simulink model "HW_2_Block_Diagram"  (R2023b)
settings: Solver=VariableStepAuto  StartTime=0.0  StopTime=15  RelTol=1e-3
values from neighbouring files (symbols this model uses):
  b = 100    [HW_2.mat]    (also in HW_2_a_Rev_1.m)
  gamma = 1    [HW_2.mat]    (also in HW_2_a_Rev_1.m)
settings Model: Creator=hkurt  LastModifiedBy=hkurt

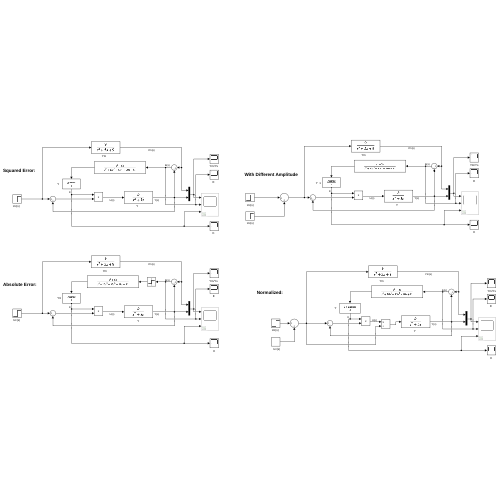
[thumbnail: Simulink's stored preview of the top-level diagram]
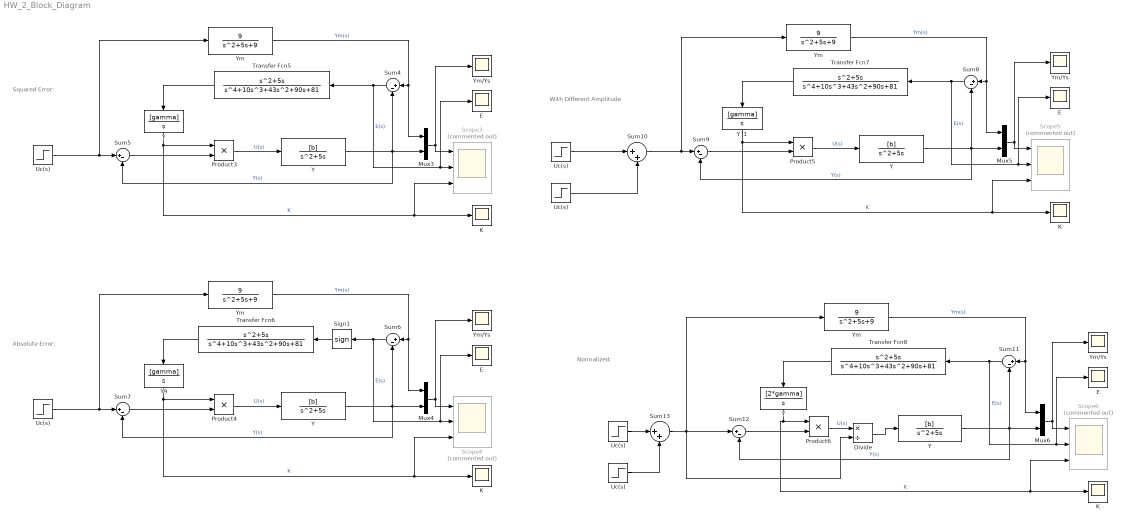
== system HW_2_Block_Diagram ==
  note: Squared Error:
  note: Absolute Error:
  note: With Different Amplitude
  note: Normalized:
  "          Uc(s)       " : Step  Time=5  After=4  SampleTime=0
  "         Uc(s)        " : Step  Time=5  After=3  SampleTime=0
  "  K  " : Scope
  "  Ym/Ys " : Scope
  " E " : Scope
  " E  " : Scope
  " K " : Scope
  " Uc(s)" : Step  SampleTime=0
  " Uc(s)  " : Step  Time=0  SampleTime=0
  " Y  " : TransferFcn  Numerator=[2*gamma]  Denominator=[1 0]
  " Y   " : TransferFcn  Numerator=[b]  Denominator=[1 5 0]
  " Ym    " : TransferFcn  Numerator=[9]  Denominator=[1 5 9]
  " Ym/Ys " : Scope
  Divide : Product  Inputs=*/
  "E " : Scope
  "E  " : Scope
  K : Scope
  "K  " : Scope
  Mux{3..6} (4 alike) : Mux  Inputs=2
  Product{3..6} (4 alike) : Product
  Scope{3..6} (4 alike) : Scope  Commented=on  NumInputPorts=3
  Sign1 : Signum
  Sum10 : Sum  Inputs=|++
  Sum{4..9,11..12} (8 alike) : Sum  Inputs=|+-
  Sum13 : Sum  Inputs=|++
  Transfer Fcn{5..8} (4 alike) : TransferFcn  Numerator=[1 5 0]  Denominator=[1 10 43 90 81]
  "Uc(s) " : Step  SampleTime=0
  "Uc(s)  " : Step  SampleTime=0
  "Y " : TransferFcn  Numerator=[b]  Denominator=[1 5 0]
  "Y  " : TransferFcn  Numerator=[gamma]  Denominator=[1 0]
  "Y   " : TransferFcn  Numerator=[b]  Denominator=[1 5 0]
  "Y    " : TransferFcn  Numerator=[b]  Denominator=[1 5 0]
  Y  1 : TransferFcn  Numerator=[gamma]  Denominator=[1 0]
  Y9 : TransferFcn  Numerator=[gamma]  Denominator=[1 0]
  "Ym  " : TransferFcn  Numerator=[9]  Denominator=[1 5 9]
  "Ym    " : TransferFcn  Numerator=[9]  Denominator=[1 5 9]
  "Ym     " : TransferFcn  Numerator=[9]  Denominator=[1 5 9]
  "Ym/Ys " : Scope
  "Ym/Ys  " : Scope
  wires:
  Mux3/1 -> "Ym/Ys "/1, Scope3/1
  "Y   "/1 -> Sum4/2, Mux3/2, Sum5/2  "Y(s)"
  Sum4/1 -> Transfer Fcn5/1, "E  "/1, Scope3/2  "E(s)"
  Transfer Fcn5/1 -> "Y  "/1
  "Y  "/1 -> "K  "/1, Scope3/3, Product3/1  "K"
  Product3/1 -> "Y   "/1  "U(s)"
  "Ym    "/1 -> Mux3/1, Sum4/1  "Ym(s)"
  Sum5/1 -> Product3/2
  "Uc(s)  "/1 -> Sum5/1, "Ym    "/1
  Mux4/1 -> "Ym/Ys  "/1, Scope4/1
  "Y "/1 -> Sum6/2, Mux4/2, Sum7/2  "Y(s)"
  Sum6/1 -> Sign1/1, "E "/1, Scope4/2  "E(s)"
  Sum7/1 -> Product4/2
  Product4/1 -> "Y "/1  "U(s)"
  Transfer Fcn6/1 -> Y9/1
  "Uc(s) "/1 -> Sum7/1, "Ym  "/1
  Y9/1 -> K/1, Scope4/3, Product4/1  "K"
  "Ym  "/1 -> Mux4/1, Sum6/1  "Ym(s)"
  Sign1/1 -> Transfer Fcn6/1
  "Y    "/1 -> Sum8/2, Mux5/2, Sum9/2  "Y(s)"
  Sum8/1 -> Transfer Fcn7/1, " E "/1, Scope5/2  "E(s)"
  Sum9/1 -> Product5/2
  Product5/1 -> "Y    "/1  "U(s)"
  Transfer Fcn7/1 -> Y  1/1
  Mux5/1 -> " Ym/Ys "/1, Scope5/1
  Y  1/1 -> " K "/1, Scope5/3, Product5/1  "K"
  "Ym     "/1 -> Mux5/1, Sum8/1  "Ym(s)"
  "         Uc(s)        "/1 -> Sum10/2
  " Uc(s)"/1 -> Sum10/1
  Sum10/1 -> "Ym     "/1, Sum9/1
  " Y   "/1 -> Sum11/2, Mux6/2, Sum12/2  "Y(s)"
  Sum11/1 -> Transfer Fcn8/1, " E  "/1, Scope6/2  "E(s)"
  Sum12/1 -> Product6/2
  Product6/1 -> Divide/1  "U(s)"
  Transfer Fcn8/1 -> " Y  "/1
  Mux6/1 -> "  Ym/Ys "/1, Scope6/1
  " Y  "/1 -> "  K  "/1, Scope6/3, Product6/1  "K"
  " Ym    "/1 -> Mux6/1, Sum11/1  "Ym(s)"
  Divide/1 -> " Y   "/1
  "          Uc(s)       "/1 -> Sum13/2
  Sum13/1 -> " Ym    "/1, Divide/2, Sum12/1
  " Uc(s)  "/1 -> Sum13/1
